simulink model "scheme"  (R2021b)
settings: Solver=FixedStepAuto  StartTime=0.0  StopTime=0.5  FixedStep=1e-4  RelTol=1e-3
libraries: fuzblock x1
settings Model: Creator=vkad  LastModifiedBy=vkad

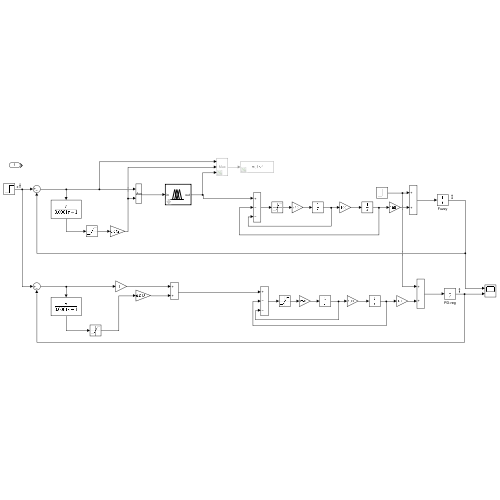
[thumbnail: Simulink's stored preview of the top-level diagram]
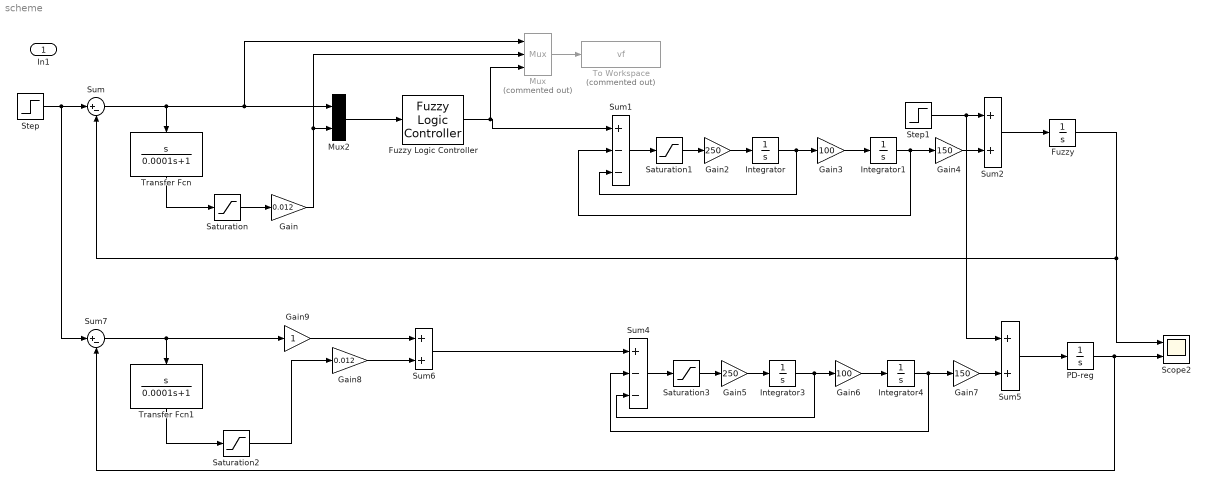
== system scheme ==
  In1 : Inport
  Fuzzy : Integrator
  Fuzzy Logic Controller : fuzblock/Fuzzy Logic  Controller  FIS='ISU_fuzzy'  OutputSampleNumber=101  DataType=double  FuzzifiedInputs=off  RuleFiringStrengths=off  RuleOutputs=off  AggregatedOutputs=off  SimulateUsing=Interpreted execution  OutOfRangeInputValueMessage=warning  NoRuleFiredMessage=warning  EmptyOutputFuzzySetMessage=warning
  Gain : Gain  Gain=0.012
  Gain2 : Gain  Gain=250
  Gain3 : Gain  Gain=100
  Gain4 : Gain  Gain=150
  Gain5 : Gain  Gain=250
  Gain6 : Gain  Gain=100
  Gain7 : Gain  Gain=150
  Gain8 : Gain  Gain=0.012
  Gain9 : Gain
  Integrator{,1,3..4} (4 alike) : Integrator
  Mux : Mux  Commented=on  Inputs=3
  Mux2 : Mux  Inputs=2
  PD-reg : Integrator
  Saturation : Saturate
  Saturation1 : Saturate  UpperLimit=0.15  LowerLimit=-0.15  LinearizeAsGain=off
  Saturation2 : Saturate
  Saturation3 : Saturate  UpperLimit=0.15  LowerLimit=-0.15  LinearizeAsGain=off
  Scope2 : Scope  NumInputPorts=2
  Step : Step  Time=0  SampleTime=0
  Step1 : Step  Time=0  After=0  SampleTime=0
  Sum : Sum  Inputs=|+-
  Sum1 : Sum  Inputs=+--
  Sum2 : Sum
  Sum4 : Sum  Inputs=+--
  Sum5 : Sum
  Sum6 : Sum
  Sum7 : Sum  Inputs=|+-
  To Workspace : ToWorkspace  Commented=on  VariableName=vf  SaveFormat=Timeseries  SampleTime=-1
  Transfer Fcn : TransferFcn  Numerator=[1 0]  Denominator=[0.0001 1]
  Transfer Fcn1 : TransferFcn  Numerator=[1 0]  Denominator=[0.0001 1]
  wires:
  Sum/1 -> Mux/1, Mux2/1, Transfer Fcn/1
  Transfer Fcn/1 -> Saturation/1
  Saturation/1 -> Gain/1
  Gain/1 -> Mux2/2, Mux/2
  Mux2/1 -> Fuzzy Logic Controller/1
  Fuzzy Logic Controller/1 -> Sum1/1, Mux/3
  Gain2/1 -> Integrator/1
  Gain3/1 -> Integrator1/1
  Integrator/1 -> Sum1/3, Gain3/1
  Integrator1/1 -> Sum1/2, Gain4/1
  Fuzzy/1 -> Sum/2, Scope2/1
  Gain4/1 -> Sum2/2
  Step1/1 -> Sum5/1, Sum2/1
  Sum2/1 -> Fuzzy/1
  Mux/1 -> To Workspace/1
  Step/1 -> Sum7/1, Sum/1
  Sum5/1 -> PD-reg/1
  Gain7/1 -> Sum5/2
  PD-reg/1 -> Scope2/2, Sum7/2
  Integrator4/1 -> Sum4/2, Gain7/1
  Integrator3/1 -> Sum4/3, Gain6/1
  Gain6/1 -> Integrator4/1
  Gain5/1 -> Integrator3/1
  Sum4/1 -> Saturation3/1
  Sum6/1 -> Sum4/1
  Gain9/1 -> Sum6/1
  Gain8/1 -> Sum6/2
  Saturation2/1 -> Gain8/1
  Transfer Fcn1/1 -> Saturation2/1
  Sum7/1 -> Transfer Fcn1/1, Gain9/1
  Saturation1/1 -> Gain2/1
  Sum1/1 -> Saturation1/1
  Saturation3/1 -> Gain5/1
